simulink model "ES239B_HwAgCorrln"  (R2013b)
settings: Solver=FixedStepDiscrete  SolverMode=SingleTasking  StartTime=0.0  StopTime=1  FixedStep=0.002  RelTol=1e-3
values from neighbouring files (symbols this model uses):
  FLTINJ_HWAGCORRLN_HWAGIDPTSIG = DataDict.Constant    [ES239B_HwAgCorrln_DataDict.m]
  HWAGCORRLNMAXSTALL_CNT_U08 = DataDict.Constant    [ES239B_HwAgCorrln_DataDict.m]
libraries: NxtrLim x2, simulink x1
settings Model: RequirementInfo="{}  %GIDa_160072ea_c0fc_4a86_8c0d_212e8c29eb83"  Creator=cz68ds  LastModifiedBy=CZ68DS
settings SolverCC: AutoInsertRateTranBlk=on  InsertRTBMode=Always
settings DataIOCC: LimitDataPoints=off  SaveFormat=Structure  ReturnWorkspaceOutputs=on
settings OptimizationCC: BlockReduction=off  InlineParams=on  ZeroExternalMemoryAtStartup=off  ZeroInternalMemoryAtStartup=off  OptimizeModelRefInitCode=on  LifeSpan=1
settings DebuggingCC: SignalInfNanChecking=error  SignalRangeChecking=warning  UnderspecifiedInitializationDetection=Simplified  MergeDetectMultiDrivingBlocksExec=error  SolverPrmCheckMsg=error  InheritedTsInSrcMsg=error  SingleTaskRateTransMsg=error  TasksWithSamePriorityMsg=error  SigSpecEnsureSampleTimeMsg=error  CheckMatrixSingularityMsg=error  ParameterUnderflowMsg=error  ParameterPrecisionLossMsg=error  ParameterTunabilityLossMsg=error  FixptConstUnderflowMsg=warning  FixptConstOverflowMsg=warning  VectorMatrixConversionMsg=error  SignalLabelMismatchMsg=error  UnconnectedInputMsg=error  UnconnectedOutputMsg=error  UnconnectedLineMsg=error  SFcnCompatibilityMsg=error  FrameProcessingCompatibilityMsg=error  UniqueDataStoreMsg=warning  BusObjectLabelMismatch=error  RootOutportRequireBusObject=error  AssertControl=DisableAll  ModelReferenceIOMsg=error  ModelReferenceVersionMismatchMessage=warning  ModelReferenceIOMismatchMessage=error  ModelReferenceDataLoggingMessage=error  StateNameClashWarn=warning  StrictBusMsg=ErrorOnBusTreatedAsVector  NonBusSignalsTreatedAsBus=error  SFUnexpectedBacktrackingDiag=error  SFInvalidInputDataAccessInChartInitDiag=error  SFNoUnconditionalDefaultTransitionDiag=error  SFTransitionOutsideNaturalParentDiag=error  SFUnconditionalTransitionShadowingDiag=error  SFUndirectedBroadcastEventsDiag=error
settings ModelReferenceCC: ModelReferenceNumInstancesAllowed=Single
settings RTWCC: SystemTargetFile=autosar.tlc  GenCodeOnly=on  TemplateMakefile=ert_default_tmf  Description=AUTOSAR  GenerateReport=on  ProcessScript=autosar_make_rtw_hook  LaunchReport=on
settings CodeAppCC: GenerateComments=off  IgnoreCustomStorageClasses=off  CustomSymbolStrType=$N$R$M  CustomSymbolStrBlkIO=$N$M  SimulinkBlockComments=off
settings STFCustomTargetCC: CodeReplacementLibrary=C89/C90 (ANSI)  ParMdlRefBuildCompliant=on  CompOptLevelCompliant=on  IncludeMdlTerminateFcn=off  CombineOutputUpdateFcns=on  SuppressErrorStatus=on  ERTFirstTimeCompliant=on  ERTCustomFileBanners=on  SupportNonFinite=off  SupportComplex=off  SupportContinuousTime=off  SupportNonInlinedSFcns=off  MATLABClassNameForMDSCustomization=Simulink.SoftwareTarget.ERTCustomization  AutosarCompliant=on  GRTInterface=off  SystemTargetFile=autosar.tlc
settings ERTTargetCC: CodeReplacementLibrary=C89/C90 (ANSI)  ConcurrentExecutionCompliant=off  IncludeMdlTerminateFcn=off  SuppressErrorStatus=on  SupportNonFinite=off  SupportComplex=off  ModelStepFunctionPrototypeControlCompliant=off  CPPClassGenCompliant=off  AutosarCompliant=on  InlinedParameterPlacement=NonHierarchical  ERTCustomFileTemplate=example_file_process.tlc  EnableUserReplacementTypes=on

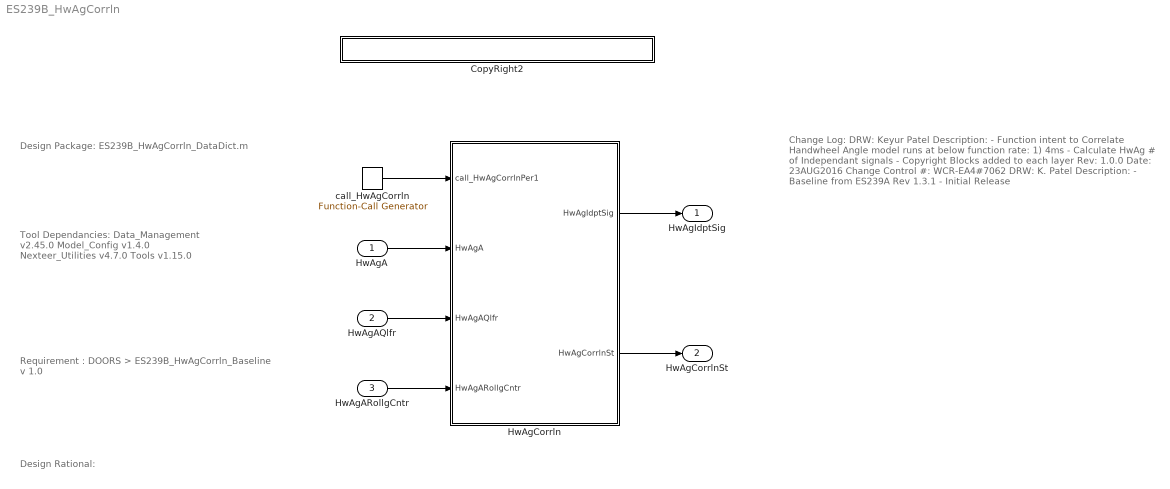
== system ES239B_HwAgCorrln ==
  note: Design Package:
      |
      | ES239B_HwAgCorrln_DataDict.m
  note: Tool Dependancies:
      |
      | Data_Management v2.45.0
      | Model_Config v1.4.0
      | Nexteer_Utilities v4.7.0
      | Tools v1.15.0
  note: Requirement :
      |
      | DOORS >
      | ES239B_HwAgCorrln_Baseline v 1.0
  note: Design Rational:
  note: Change Log:
      |
      | DRW: Keyur Patel
      | Description:
      | - Function intent to Correlate Handwheel Angle
      |    model runs at below function rate:
      |       1) 4ms - Calculate HwAg # of Independant signals
      | - Copyright Blocks added to each layer
      |
      | Rev: 1.0.0
      | Date: 23AUG2016
      | Change Control #: WCR-EA4#7062
      | DRW: K. Patel
      | Description:
      | - Baseline from ES239A Rev 1.3.1 - Initial Release
  HwAgA : Inport
  HwAgAQlfr : Inport  Port=2
  HwAgARollgCntr : Inport  Port=3
  CopyRight2 : Subsystem  Description=|  mask(Copyright Information){none=on}
      | Copyright info block.                                               
      |                                                                     
      | Place copyright information at the top of every subsystem in design.
      mask prompts: none "No parameters"
      mask help: Place copyright information at the top of every subsystem in design.
      mask Display:
      | NxtrConf = 'Nexteer Confidential';
      | 
      | sys = bdroot; %handle for the current model ("system")
      | first = get_param(sys,'Created');
      | first = first(end-3:end);  %year is last four digits
      | 
      | last = get_param(sys,'LastModifiedDate');
      | if isempty(last)
      |     last = datestr(now,'yyyy');
      | else
      |     last = last(end-3:end);
      | end
      | 
      | if strcmp(first,last)
      |     fprintf('%s -- Copyright %s Nexteer',NxtrConf,first)
      | else
      |     fprintf('%s -- %s%s- %s Nexteer',NxtrConf,char(169),first,last)
      | end
  HwAgCorrln : Subsystem  RequirementInfo="{}  %GIDa_007a48a9_e344_4cef_a432_d99ae24057fc"
      settings: AttributesFormatString=%<Tag>
  call_HwAgCorrln : simulink/Ports & Subsystems/Function-Call Generator  sample_time=0.004  numberOfIterations=1
      settings: AttributesFormatString=%<sample_time>
  HwAgIdptSig : Outport
  HwAgCorrlnSt : Outport  Port=2
  wires:
  call_HwAgCorrln/1 -> HwAgCorrln/1(call_HwAgCorrlnPer1)
  HwAgCorrln/1(HwAgIdptSig) -> HwAgIdptSig/1
  HwAgCorrln/2(HwAgCorrlnSt) -> HwAgCorrlnSt/1
  HwAgA/1 -> HwAgCorrln/2(HwAgA)
  HwAgAQlfr/1 -> HwAgCorrln/3(HwAgAQlfr)
  HwAgARollgCntr/1 -> HwAgCorrln/4(HwAgARollgCntr)

== system ES239B_HwAgCorrln/CopyRight2 ==

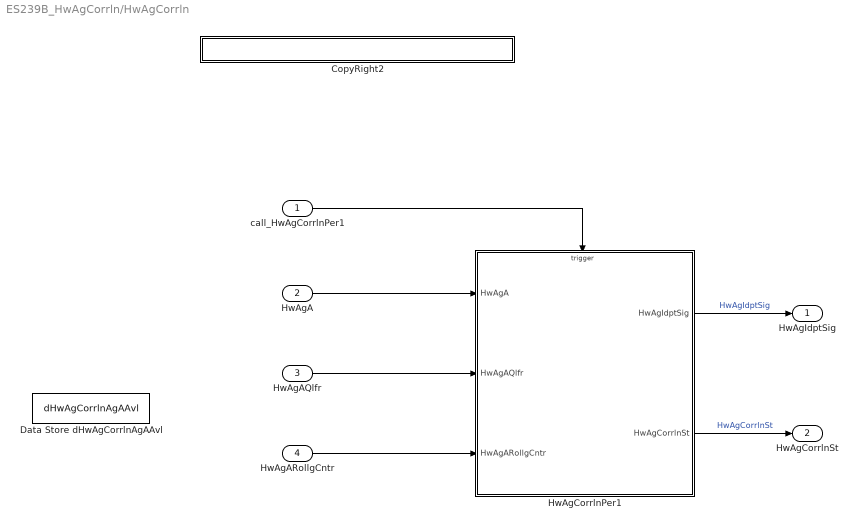
== system ES239B_HwAgCorrln/HwAgCorrln ==
  call_HwAgCorrlnPer1 : Inport
  HwAgA : Inport  Port=2
  HwAgAQlfr : Inport  Port=3
  HwAgARollgCntr : Inport  Port=4
  CopyRight2 : Subsystem  Description=|  mask(Copyright Information){none=on}
      | Copyright info block.                                               
      |                                                                     
      | Place copyright information at the top of every subsystem in design.
      mask prompts: none "No parameters"
      mask help: Place copyright information at the top of every subsystem in design.
      mask Display:
      | NxtrConf = 'Nexteer Confidential';
      | 
      | sys = bdroot; %handle for the current model ("system")
      | first = get_param(sys,'Created');
      | first = first(end-3:end);  %year is last four digits
      | 
      | last = get_param(sys,'LastModifiedDate');
      | if isempty(last)
      |     last = datestr(now,'yyyy');
      | else
      |     last = last(end-3:end);
      | end
      | 
      | if strcmp(first,last)
      |     fprintf('%s -- Copyright %s Nexteer',NxtrConf,first)
      | else
      |     fprintf('%s -- %s%s- %s Nexteer',NxtrConf,char(169),first,last)
      | end
  Data Store dHwAgCorrlnAgAAvl : DataStoreMemory  DataStoreName=dHwAgCorrlnAgAAvl  StateMustResolveToSignalObject=on
  HwAgCorrlnPer1 : Subsystem  Tag=0.002  TreatAsAtomicUnit=on
  HwAgIdptSig : Outport
  HwAgCorrlnSt : Outport  Port=2
  wires:
  HwAgCorrlnPer1/1(HwAgIdptSig) -> HwAgIdptSig/1  "HwAgIdptSig"
  call_HwAgCorrlnPer1/1 -> HwAgCorrlnPer1/Trigger
  HwAgA/1 -> HwAgCorrlnPer1/1(HwAgA)
  HwAgAQlfr/1 -> HwAgCorrlnPer1/2(HwAgAQlfr)
  HwAgARollgCntr/1 -> HwAgCorrlnPer1/3(HwAgARollgCntr)
  HwAgCorrlnPer1/2(HwAgCorrlnSt) -> HwAgCorrlnSt/1  "HwAgCorrlnSt"

== system ES239B_HwAgCorrln/HwAgCorrln/CopyRight2 ==

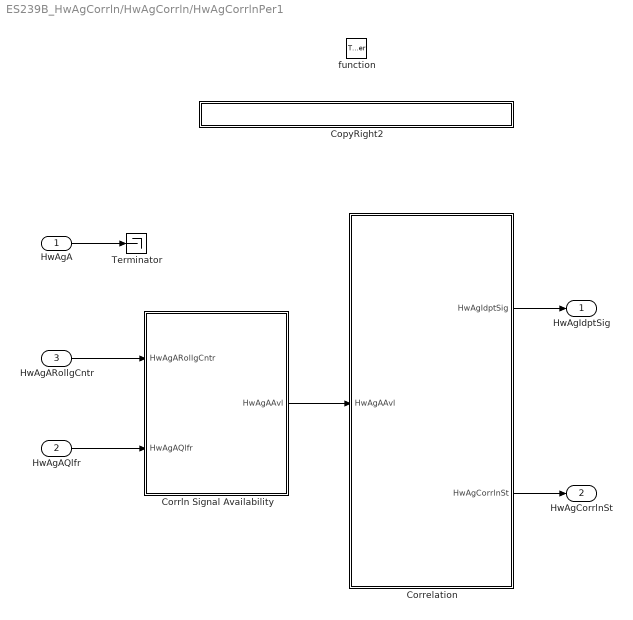
== system ES239B_HwAgCorrln/HwAgCorrln/HwAgCorrlnPer1 ==
  HwAgA : Inport
  HwAgAQlfr : Inport  Port=2
  HwAgARollgCntr : Inport  Port=3
  function : TriggerPort  TriggerType=function-call
  CopyRight2 : Subsystem  Description=|  mask(Copyright Information){none=on}
      | Copyright info block.                                               
      |                                                                     
      | Place copyright information at the top of every subsystem in design.
      mask prompts: none "No parameters"
      mask help: Place copyright information at the top of every subsystem in design.
      mask Display:
      | NxtrConf = 'Nexteer Confidential';
      | 
      | sys = bdroot; %handle for the current model ("system")
      | first = get_param(sys,'Created');
      | first = first(end-3:end);  %year is last four digits
      | 
      | last = get_param(sys,'LastModifiedDate');
      | if isempty(last)
      |     last = datestr(now,'yyyy');
      | else
      |     last = last(end-3:end);
      | end
      | 
      | if strcmp(first,last)
      |     fprintf('%s -- Copyright %s Nexteer',NxtrConf,first)
      | else
      |     fprintf('%s -- %s%s- %s Nexteer',NxtrConf,char(169),first,last)
      | end
  "Correlation " : Subsystem
  Corrln Signal Availability : Subsystem  RequirementInfo={'linktype_rmi_doors' '00011b4c (/ESG Group/FDD Module Requirements/EA4 Specific/ES239B_HwAgCorrln)' '#ES239B_20' 'true' 'REQ:ES239B_20' '' } %GIDa_1a8fc132_5d68_403f_a6c5_f3af5bb08ac2
  Terminator : Terminator
  HwAgIdptSig : Outport
  HwAgCorrlnSt : Outport  Port=2
  wires:
  HwAgAQlfr/1 -> Corrln Signal Availability/2(HwAgAQlfr)
  HwAgARollgCntr/1 -> Corrln Signal Availability/1(HwAgARollgCntr)
  "Correlation "/1(HwAgIdptSig) -> HwAgIdptSig/1
  "Correlation "/2(HwAgCorrlnSt) -> HwAgCorrlnSt/1
  Corrln Signal Availability/1(HwAgAAvl) -> "Correlation "/1(HwAgAAvl)
  HwAgA/1 -> Terminator/1

== system ES239B_HwAgCorrln/HwAgCorrln/HwAgCorrlnPer1/CopyRight2 ==

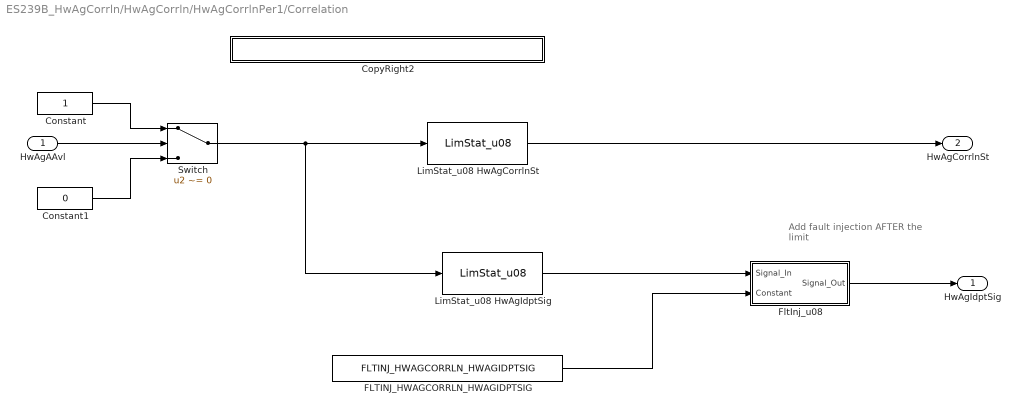
== system ES239B_HwAgCorrln/HwAgCorrln/HwAgCorrlnPer1/Correlation  ==
  note: Add fault injection
      | AFTER the limit
  HwAgAAvl : Inport
  Constant : Constant  RequirementInfo={} %GIDa_4a8a31dd_b787_4382_8d5f_cc6712202a6c  OutDataTypeStr=uint8
  Constant1 : Constant  RequirementInfo={} %GIDa_b2b38bb4_e4b7_417a_8236_7766f3a066e5  Value=0  OutDataTypeStr=uint8
  CopyRight2 : Subsystem  Description=|  mask(Copyright Information){none=on}
      | Copyright info block.                                               
      |                                                                     
      | Place copyright information at the top of every subsystem in design.
      mask prompts: none "No parameters"
      mask help: Place copyright information at the top of every subsystem in design.
      mask Display:
      | NxtrConf = 'Nexteer Confidential';
      | 
      | sys = bdroot; %handle for the current model ("system")
      | first = get_param(sys,'Created');
      | first = first(end-3:end);  %year is last four digits
      | 
      | last = get_param(sys,'LastModifiedDate');
      | if isempty(last)
      |     last = datestr(now,'yyyy');
      | else
      |     last = last(end-3:end);
      | end
      | 
      | if strcmp(first,last)
      |     fprintf('%s -- Copyright %s Nexteer',NxtrConf,first)
      | else
      |     fprintf('%s -- %s%s- %s Nexteer',NxtrConf,char(169),first,last)
      | end
  FLTINJ_HWAGCORRLN_HWAGIDPTSIG : Constant  RequirementInfo={} %GIDa_dcd4ef43_6b76_41ba_bfae_1fba77b8b422  Value=FLTINJ_HWAGCORRLN_HWAGIDPTSIG
  FltInj_u08 : Subsystem  RequirementInfo={} %GIDa_81dbf112_3f37_469e_8630_4577ca85f452  TreatAsAtomicUnit=on  VariantControl=FltInj_sim  mask(Fault_Injection){}
      mask help: Fault Injection is a simulation only block for EA3 programs.
  LimStat_u08 HwAgCorrlnSt : NxtrLim/LimStat_u08  LoLim=HwAgIdptSig.EngMin  HiLim=HwAgIdptSig.EngMax
      settings: AttributesFormatString=|
      | Low Limit: %<LoLim> :0
      | High Limit:%<HiLim> :1
  LimStat_u08 HwAgIdptSig : NxtrLim/LimStat_u08  LoLim=HwAgIdptSig.EngMin  HiLim=HwAgIdptSig.EngMax
      settings: AttributesFormatString=|
      | Low Limit: %<LoLim> : 0
      | High Limit:%<HiLim>  : 2
  Switch : Switch  RequirementInfo={'linktype_rmi_doors' '00011b4c (/ESG Group/FDD Module Requirements/EA4 Specific/ES239B_HwAgCorrln)' '#ES239B_21' 'true' 'REQ:ES239B_21' '' ; 'linktype_rmi_doors' '00011b4c (/ESG Group/FDD Module Requirements/EA4 Specific/ES239B_HwAgCorrln)' '#ES239B_22' 'true' 'REQ:ES239B_22' '' } %GIDa_8ce41c67_22af_43de_9e7f_1d6b6d9d200a  Criteria=u2 ~= 0
  HwAgIdptSig : Outport
  HwAgCorrlnSt : Outport  Port=2
  wires:
  LimStat_u08 HwAgIdptSig/1 -> FltInj_u08/1(Signal_In)
  LimStat_u08 HwAgCorrlnSt/1 -> HwAgCorrlnSt/1
  FltInj_u08/1(Signal_Out) -> HwAgIdptSig/1
  FLTINJ_HWAGCORRLN_HWAGIDPTSIG/1 -> FltInj_u08/2(Constant)
  HwAgAAvl/1 -> Switch/2
  Constant/1 -> Switch/1
  Constant1/1 -> Switch/3
  Switch/1 -> LimStat_u08 HwAgIdptSig/1, LimStat_u08 HwAgCorrlnSt/1

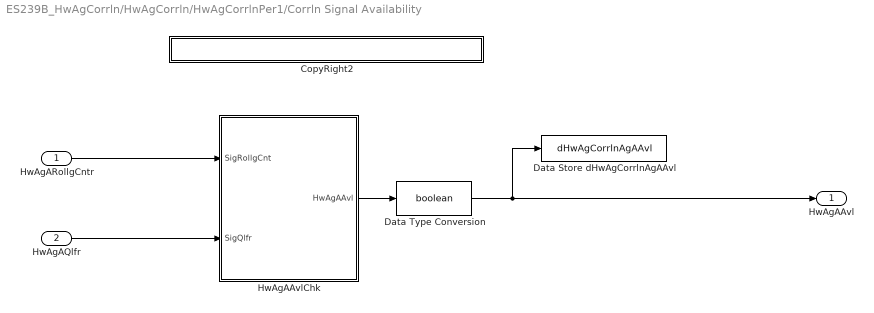
== system ES239B_HwAgCorrln/HwAgCorrln/HwAgCorrlnPer1/Corrln Signal Availability ==
  HwAgARollgCntr : Inport
  HwAgAQlfr : Inport  Port=2
  CopyRight2 : Subsystem  Description=|  mask(Copyright Information){none=on}
      | Copyright info block.                                               
      |                                                                     
      | Place copyright information at the top of every subsystem in design.
      mask prompts: none "No parameters"
      mask help: Place copyright information at the top of every subsystem in design.
      mask Display:
      | NxtrConf = 'Nexteer Confidential';
      | 
      | sys = bdroot; %handle for the current model ("system")
      | first = get_param(sys,'Created');
      | first = first(end-3:end);  %year is last four digits
      | 
      | last = get_param(sys,'LastModifiedDate');
      | if isempty(last)
      |     last = datestr(now,'yyyy');
      | else
      |     last = last(end-3:end);
      | end
      | 
      | if strcmp(first,last)
      |     fprintf('%s -- Copyright %s Nexteer',NxtrConf,first)
      | else
      |     fprintf('%s -- %s%s- %s Nexteer',NxtrConf,char(169),first,last)
      | end
  Data Store dHwAgCorrlnAgAAvl : DataStoreWrite  RequirementInfo={} %GIDa_69226d58_3222_4378_b58d_6edad87bfcb0  DataStoreName=dHwAgCorrlnAgAAvl
  Data Type Conversion : DataTypeConversion  OutDataTypeStr=boolean
  HwAgAAvlChk : Subsystem  RequirementInfo={} %GIDa_afd08659_04a6_48fb_a6d8_df09dfc0c7b5  TreatAsAtomicUnit=on
  HwAgAAvl : Outport
  wires:
  HwAgAQlfr/1 -> HwAgAAvlChk/2(SigQlfr)
  HwAgARollgCntr/1 -> HwAgAAvlChk/1(SigRollgCnt)
  HwAgAAvlChk/1(HwAgAAvl) -> Data Type Conversion/1
  Data Type Conversion/1 -> Data Store dHwAgCorrlnAgAAvl/1, HwAgAAvl/1

== system ES239B_HwAgCorrln/HwAgCorrln/HwAgCorrlnPer1/Correlation /CopyRight2 ==

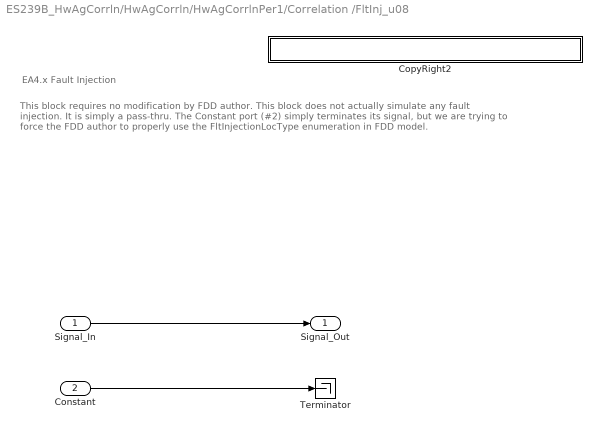
== system ES239B_HwAgCorrln/HwAgCorrln/HwAgCorrlnPer1/Correlation /FltInj_u08 ==
  note: This block requires no modification by FDD author.
      |
      | This block does not actually simulate any fault injection.  It is simply a pass-thru.
      |
      | The Constant port (#2) simply terminates its signal, but we are trying to force the FDD author
      | to properly use the FltInjectionLocType enumeration in FDD model.
  note: EA4.x Fault Injection
  Signal_In : Inport
  Constant : Inport  Port=2
  CopyRight2 : Subsystem  Description=|  mask(Copyright Information){none=on}
      | Copyright info block.                                               
      |                                                                     
      | Place copyright information at the top of every subsystem in design.
      mask prompts: none "No parameters"
      mask help: Place copyright information at the top of every subsystem in design.
      mask Display:
      | NxtrConf = 'Nexteer Confidential';
      | 
      | sys = bdroot; %handle for the current model ("system")
      | first = get_param(sys,'Created');
      | first = first(end-3:end);  %year is last four digits
      | 
      | last = get_param(sys,'LastModifiedDate');
      | if isempty(last)
      |     last = datestr(now,'yyyy');
      | else
      |     last = last(end-3:end);
      | end
      | 
      | if strcmp(first,last)
      |     fprintf('%s -- Copyright %s Nexteer',NxtrConf,first)
      | else
      |     fprintf('%s -- %s%s- %s Nexteer',NxtrConf,char(169),first,last)
      | end
  Terminator : Terminator
  Signal_Out : Outport
  wires:
  Signal_In/1 -> Signal_Out/1
  Constant/1 -> Terminator/1

== system ES239B_HwAgCorrln/HwAgCorrln/HwAgCorrlnPer1/Corrln Signal Availability/CopyRight2 ==

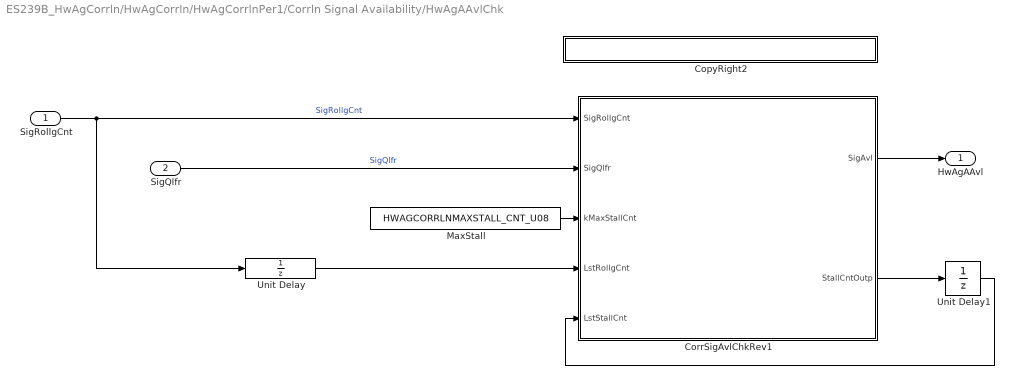
== system ES239B_HwAgCorrln/HwAgCorrln/HwAgCorrlnPer1/Corrln Signal Availability/HwAgAAvlChk ==
  SigRollgCnt : Inport  OutDataTypeStr=uint8
  SigQlfr : Inport  Port=2  OutDataTypeStr=uint8
  CopyRight2 : Subsystem  Description=|  mask(Copyright Information){none=on}
      | Copyright info block.                                               
      |                                                                     
      | Place copyright information at the top of every subsystem in design.
      mask prompts: none "No parameters"
      mask help: Place copyright information at the top of every subsystem in design.
      mask Display:
      | NxtrConf = 'Nexteer Confidential';
      | 
      | sys = bdroot; %handle for the current model ("system")
      | first = get_param(sys,'Created');
      | first = first(end-3:end);  %year is last four digits
      | 
      | last = get_param(sys,'LastModifiedDate');
      | if isempty(last)
      |     last = datestr(now,'yyyy');
      | else
      |     last = last(end-3:end);
      | end
      | 
      | if strcmp(first,last)
      |     fprintf('%s -- Copyright %s Nexteer',NxtrConf,first)
      | else
      |     fprintf('%s -- %s%s- %s Nexteer',NxtrConf,char(169),first,last)
      | end
  CorrSigAvlChkRev1 : Stateflow chart  TreatAsAtomicUnit=on
  MaxStall : Constant  Value=HWAGCORRLNMAXSTALL_CNT_U08
      settings: AttributesFormatString=%<Value> = 200
  Unit Delay : UnitDelay  SampleTime=-1  StateName=HwAgARollgCntPrev  StateMustResolveToSignalObject=on
      settings: AttributesFormatString=|
      | State Variable:
      | %<StateName>
  Unit Delay1 : UnitDelay  SampleTime=-1  StateName=HwAgAStallCntPrev  StateMustResolveToSignalObject=on
      settings: AttributesFormatString=|
      | State Variable:
      | %<StateName>
  HwAgAAvl : Outport
  wires:
  SigRollgCnt/1 -> CorrSigAvlChkRev1/1(SigRollgCnt), Unit Delay/1  "SigRollgCnt"
  SigQlfr/1 -> CorrSigAvlChkRev1/2(SigQlfr)  "SigQlfr"
  Unit Delay/1 -> CorrSigAvlChkRev1/4(LstRollgCnt)
  CorrSigAvlChkRev1/2(StallCntOutp) -> Unit Delay1/1
  Unit Delay1/1 -> CorrSigAvlChkRev1/5(LstStallCnt)
  CorrSigAvlChkRev1/1(SigAvl) -> HwAgAAvl/1
  MaxStall/1 -> CorrSigAvlChkRev1/3(kMaxStallCnt)

== system ES239B_HwAgCorrln/HwAgCorrln/HwAgCorrlnPer1/Correlation /FltInj_u08/CopyRight2 ==

== system ES239B_HwAgCorrln/HwAgCorrln/HwAgCorrlnPer1/Corrln Signal Availability/HwAgAAvlChk/CopyRight2 ==

== stateflow chart ES239B_HwAgCorrln/HwAgCorrln/HwAgCorrlnPer1/Corrln Signal Availability/HwAgAAvlChk/CorrSigAvlChkRev1 ==
  note: SigAvl
      | False = 0
      | Pass = 1
  note: SigQlfr
      | 0 = No Result
      | 1 = Pass
      | 2 = Fail
  (default) -> (junction 2)
  (junction 2) -> (junction 4) [order 1] : [SigRollgCnt ==LstRollgCnt]
  (junction 4) -> (junction 7) [order 2] : {
      | StallCntOutp = LstStallCnt +1;
      | }
  (junction 2) -> (junction 3) [order 2]
  (junction 4) -> (junction 7) [order 1] : [LstStallCnt == 255]
      | {
      | StallCntOutp = 255;
      | }
  (junction 3) -> (junction 7) : {
      | StallCntOutp = 0;
      | }
  (junction 7) -> (junction 10)
  (junction 10) -> (junction 12) [order 1] : [StallCntOutp >=kMaxStallCnt]
  (junction 10) -> (junction 14) [order 2]
  (junction 12) -> (junction 17)
  (junction 14) -> (junction 17) [order 2]
  (junction 14) -> (junction 16) [order 1] : [SigQlfr<2]
  (junction 17) -> (junction 29) : {
      | SigAvl =0;
      | }
  (junction 16) -> (junction 29) : {
      | SigAvl = 1;
      | }
  data: SigRollgCnt input; SigQlfr input; kMaxStallCnt input; SigAvl output uint8; LstRollgCnt input uint8; LstStallCnt input uint8; StallCntOutp output uint8
